simulink model "TST_EnumTypesStateflow"  (Simulink 7.4)
settings: Solver=FixedStepDiscrete  StartTime=0.0  StopTime=10.0  FixedStep=0.02  RelTol=1e-3
undefined symbols (not defined in the file): DIL_VmmGsFcsCommandsMessage_LatApModeCmd, DIL_VmmGsFcsCommandsMessage_LongApModeCmd
settings Model: Creator=kharthforeign  LastModifiedBy=kharthforeign  BufferReuse=off
settings DataIOCC: SaveOutput=off  SignalLogging=off  SaveTime=off
settings OptimizationCC: BlockReduction=off  ConditionallyExecuteInputs=off  OptimizeBlockIOStorage=off  BufferReuse=off  ExpressionFolding=off  LocalBlockOutputs=off  InitFltsAndDblsToZero=on

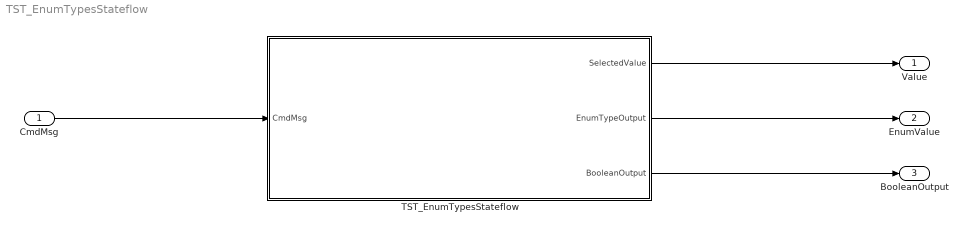
== system TST_EnumTypesStateflow ==
  CmdMsg : Inport  UseBusObject=on  OutDataType=fixdt(1, 16)  OutScaling=2^0  BusOutputAsStruct=on
      settings: BusObject=DIL_VmmGsFcsCommandsMessage_Data
  TST_EnumTypesStateflow : Subsystem  TreatAsAtomicUnit=on
  Value : Outport  PortDimensions=1  DataType=double  OutDataType=fixdt(1, 16)  OutScaling=2^0  OutDataTypeStr=double
  EnumValue : Outport  Port=2  PortDimensions=1  DataType=Specify via dialog  OutDataType=Enum: DIL_VmmGsFcsCommandsMessage_LatApModeCmd  OutDataTypeStr=Enum: DIL_VmmGsFcsCommandsMessage_LatApModeCmd
  BooleanOutput : Outport  Port=3  PortDimensions=1  DataType=boolean  OutDataType=fixdt(1, 16)  OutScaling=2^0  OutDataTypeStr=boolean
  wires:
  CmdMsg/1 -> TST_EnumTypesStateflow/1(CmdMsg)
  TST_EnumTypesStateflow/1(SelectedValue) -> Value/1
  TST_EnumTypesStateflow/2(EnumTypeOutput) -> EnumValue/1
  TST_EnumTypesStateflow/3(BooleanOutput) -> BooleanOutput/1

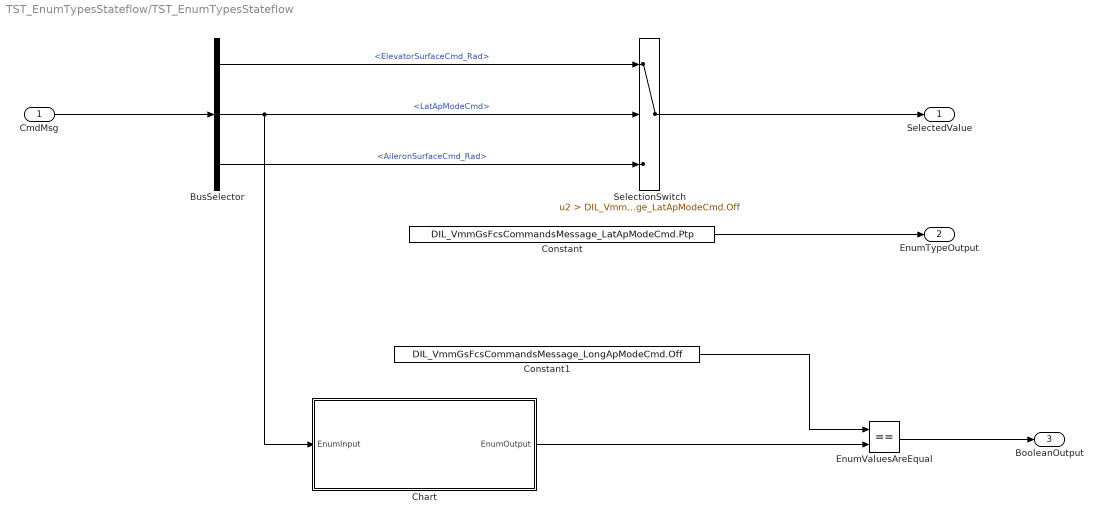
== system TST_EnumTypesStateflow/TST_EnumTypesStateflow ==
  CmdMsg : Inport  UseBusObject=on  OutDataType=fixdt(1, 16)  OutScaling=2^0
      settings: BusObject=DIL_VmmGsFcsCommandsMessage_Data
  BusSelector : BusSelector  OutputSignals=ElevatorSurfaceCmd_Rad,LatApModeCmd,AileronSurfaceCmd_Rad
  Chart : Stateflow chart
  Constant : Constant  Value=DIL_VmmGsFcsCommandsMessage_LatApModeCmd.Ptp  OutDataTypeMode=Specify via dialog  OutDataType=Enum: DIL_VmmGsFcsCommandsMessage_LatApModeCmd  ConRadixGroup=Best Precision: Vector-wise  OutDataTypeStr=Enum: DIL_VmmGsFcsCommandsMessage_LatApModeCmd
  Constant1 : Constant  Value=DIL_VmmGsFcsCommandsMessage_LongApModeCmd.Off  OutDataType=Enum: DIL_VmmGsFcsCommandsMessage_LatApModeCmd  ConRadixGroup=Best Precision: Vector-wise
  EnumValuesAreEqual : RelationalOperator  Operator===  LogicOutDataTypeMode=boolean  LogicDataType=fixdt(0, 8)  OutDataTypeStr=boolean
  SelectionSwitch : Switch  Criteria=u2 > Threshold  Threshold=DIL_VmmGsFcsCommandsMessage_LatApModeCmd.Off  OutDataType=fixdt(1, 16)  OutScaling=2^0
  SelectedValue : Outport  PortDimensions=1  DataType=double  OutDataType=fixdt(1, 16)  OutScaling=2^0  OutDataTypeStr=double
  EnumTypeOutput : Outport  Port=2  PortDimensions=1  DataType=Specify via dialog  OutDataType=Enum: DIL_VmmGsFcsCommandsMessage_LatApModeCmd  OutDataTypeStr=Enum: DIL_VmmGsFcsCommandsMessage_LatApModeCmd
  BooleanOutput : Outport  Port=3  PortDimensions=1  DataType=boolean  OutDataType=fixdt(1, 16)  OutScaling=2^0  OutDataTypeStr=boolean
  wires:
  CmdMsg/1 -> BusSelector/1
  SelectionSwitch/1 -> SelectedValue/1
  BusSelector/1 -> SelectionSwitch/1  "<ElevatorSurfaceCmd_Rad>"
  BusSelector/3 -> SelectionSwitch/3  "<AileronSurfaceCmd_Rad>"
  BusSelector/2 -> SelectionSwitch/2, Chart/1(EnumInput)  "<LatApModeCmd>"
  Constant/1 -> EnumTypeOutput/1
  Constant1/1 -> EnumValuesAreEqual/1
  Chart/1(EnumOutput) -> EnumValuesAreEqual/2
  EnumValuesAreEqual/1 -> BooleanOutput/1

== stateflow chart TST_EnumTypesStateflow/Chart ==
  state Ping
  state Pong
    entry:
    EnumOutput = ...
    DIL_VmmGsFcsCommandsMessage_LongApModeCmd.Altitude;
  (default) -> Ping
  Ping -> Pong : [EnumInput == ...
      |    DIL_VmmGsFcsCommandsMessage_LatApModeCmd.BankHeading]
  data: EnumInput input Enum: DIL_VmmGsFcsCommandsMessage_LatApModeCmd; EnumOutput output Enum: DIL_VmmGsFcsCommandsMessage_LongApModeCmd =DIL_VmmGsFcsCommandsMessage_LongApModeCmd.Off
